simulink model "SOC_Estimation"  (R2022b)
settings: configuration reference "BMS_Sw_CodeGenConfig" (kept outside this file)
undefined symbols (not defined in the file): battery_sli_rtmsupport, BatteryNN, BMS_State_Enum, C1_mat, c_sqrt, DiscIntNeverNeededParam, dV0_mat, gcbh, n, Np_Module, Ns_Module, NumModules, SOCInit, Wc, Wm, x0
libraries: simulink x1
(part 1 of 2)
settings Model: DataDictionary=DD_SOC_Estimation.sldd  ExtModeTrigDuration=5  Creator=cpatel  LastModifiedBy=cpatel
settings ConfigSetRef: SourceName=BMS_Sw_CodeGenConfig

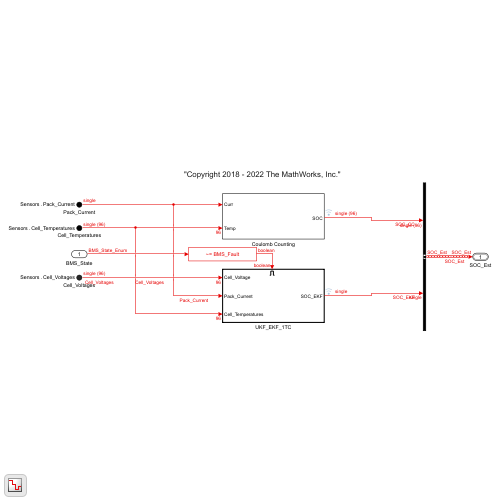
[thumbnail: Simulink's stored preview of the top-level diagram]
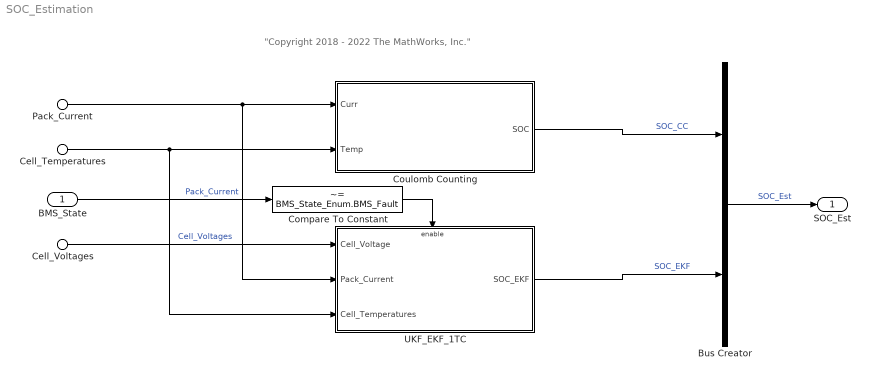
== system SOC_Estimation ==
  note: "Copyright 2018 - 2022 The MathWorks, Inc."
  BMS_State : Inport  OutDataTypeStr=Enum: BMS_State_Enum
  Cell_Voltages : Inport  Port=2  PortName=Sensors  Element=Cell_Voltages
  Pack_Current : Inport  Port=2  PortName=Sensors  Element=Pack_Current
  Cell_Temperatures : Inport  Port=2  PortName=Sensors  Element=Cell_Temperatures
  Bus Creator : BusCreator  Inputs=2  OutDataTypeStr=Bus: SOC_Est  NonVirtualBus=on
      settings: InheritFromInputs=off
  Compare To Constant : simulink/Logic and Bit Operations/Compare To Constant  relop=~=  const=BMS_State_Enum.BMS_Fault  OutDataTypeStr=boolean
  Coulomb Counting : Subsystem  VariantControl=SocAlgo==1
  UKF_EKF_1TC : Subsystem  VariantControl=CellType==1
  SOC_Est : Outport  OutDataTypeStr=Bus: SOC_Est  SampleTime=[0.10000000000000001,0]  VectorParamsAs1DForOutWhenUnconnected=off  BusOutputAsStruct=on
  wires:
  Cell_Voltages/1 -> UKF_EKF_1TC/1(Cell_Voltage)  "Cell_Voltages"
  Bus Creator/1 -> SOC_Est/1  "SOC_Est"
  Coulomb Counting/1(SOC) -> Bus Creator/1  "SOC_CC"
  UKF_EKF_1TC/1(SOC_EKF) -> Bus Creator/2  "SOC_EKF"
  BMS_State/1 -> Compare To Constant/1
  Compare To Constant/1 -> UKF_EKF_1TC/Enable
  Pack_Current/1 -> UKF_EKF_1TC/2(Pack_Current), Coulomb Counting/1(Curr)  "Pack_Current"
  Cell_Temperatures/1 -> Coulomb Counting/2(Temp), UKF_EKF_1TC/3(Cell_Temperatures)

== system SOC_Estimation/Coulomb Counting ==
  Curr : Inport
  Temp : Inport  Port=2
  1-D Lookup Table : Lookup_n-D  NumberOfTableDimensions=1  BreakpointsForDimension1=single(BatteryNN(1).T_vec)  Table=single(BatteryNN(1).AH)*Np_Module  InternalRulePriority=Speed  RndMeth=Simplest
  Discrete-Time Integrator : DiscreteIntegrator  InitialCondition=ones(1,NumModules*Ns_Module)*single(SOCInit)  SampleTime=-1  LimitOutput=on  UpperSaturationLimit=1  LowerSaturationLimit=0  ICPrevOutput=DiscIntNeverNeededParam  ICPrevScaledInput=DiscIntNeverNeededParam
  Divide : Product  Inputs=*/
  Gain : Gain  Gain=single(1/3600)
  SOC : Outport  VectorParamsAs1DForOutWhenUnconnected=off
  wires:
  Discrete-Time Integrator/1 -> SOC/1
  Curr/1 -> Gain/1
  Gain/1 -> Divide/1
  Divide/1 -> Discrete-Time Integrator/1
  1-D Lookup Table/1 -> Divide/2  "Capacity"
  Temp/1 -> 1-D Lookup Table/1

== system SOC_Estimation/UKF_EKF_1TC ==
  note: SOC Blocks have been modified from original library block from Simscape Battery
      | to use Single Data Type
  Cell_Voltage : Inport
  Pack_Current : Inport  Port=2
  Cell_Temperatures : Inport  Port=3
  Enable : EnablePort
  Constant : Constant  Value=single(0.98)
  Constant1 : Constant  Value=single(0.15)
  SOC EKF Estimator (Adaptive Kalman Filter) : Subsystem  LoadFcn=battery_sli_rtmsupport( 'loadfcn', gcbh );  TreatAsAtomicUnit=on  mask(SOC Estimator (Adaptive Kalman Filter)){filterType=Extended Kalman filter, alpha=1, beta=2, kappa=0, Q=|, R=single(0.001), P0=single([1e-2 0 0; 0 1 0; 0 0 1e-8]), Ts=-1, SOC_vec=single(BatteryNN.SOC_vec'), T_vec=single(BatteryNN.T_vec), R1_mat=single(1e-05*ones(11,6)), tau1_mat=single(30*ones(11,6)), V0_mat=single(BatteryNN.V0_mat), AH=single(BatteryNN.AH(1)*Np_Module)}
      mask Q=|
      | single([1e-5 0 0;
      | 0 5e-1 0;0 0 1e-6])
      mask prompts: filterType "physmod:battery:library:comments:control:BatteryEstimators:FilterType_MP"; alpha "physmod:battery:library:comments:control:BatteryEstimators:Alpha_MP"; beta "physmod:battery:library:comments:control:BatteryEstimators:Beta_MP"; kappa "physmod:battery:library:comments:control:BatteryEstimators:Kappa_MP"; Q "physmod:battery:library:comments:control:BatteryEstimators:CovarianceOfTheProcessNoiseQ_MP"; R "physmod:battery:library:comments:control:BatteryEstimators:CovarianceOfTheMeasurementNoiseR_MP"; P0 "physmod:battery:library:comments:control:BatteryEstimators:InitialStateErrorCovarianceP0_MP"; Ts "physmod:battery:library:comments:control:BatteryEstimators:SampleTime1ForInherited_MP"; SOC_vec "physmod:battery:library:comments:control:BatteryEstimators:VectorOfStateofchargeValuesSOC_MP"; T_vec "physmod:battery:library:comments:control:BatteryEstimators:VectorOfTemperaturesT_MP"; R1_mat "physmod:battery:library:comments:control:BatteryEstimators:FirstPolarizationResistanceR1SOCT_MP"; tau1_mat "physmod:battery:library:comments:control:BatteryEstimators:FirstTimeConstantTau1SOCT_MP"; V0_mat "physmod:battery:library:comments:control:BatteryEstimators:NoloadVoltageV0SOCT_MP"; AH "physmod:battery:library:comments:control:BatteryEstimators:CellCapacityAH_MP"
      mask help: physmod:battery:library:comments:control:BatteryEstimators:SOCEstimatorAdaptiveKalmanFilter_MD
      mask init:
      | [C1_mat,dV0_mat,m,n,Wm,Wc,c_sqrt] = battery.mask.initializeKalmanFilter(filterType,tau1_mat,R1_mat,V0_mat,SOC_vec,T_vec,P0,R,Q,alpha,beta,kappa,Ts,AH); %#ok
      settings: CopyFcn=battery_sli_rtmsupport( 'copyfcn', gcbh );  DeleteFcn=battery_sli_rtmsupport( 'deletefcn', gcbh );  ModelCloseFcn=battery_sli_rtmsupport( 'modelclosefcn', gcbh );  PostSaveFcn=battery_sli_rtmsupport( 'postsavefcn', gcbh );  PreCopyFcn=battery_sli_rtmsupport( 'precopyfcn', gcbh );  OpenFcn=battery_sli_rtmsupport( 'openfcn', gcbh );  CloseFcn=battery_sli_rtmsupport( 'closefcn', gcbh );  PreDeleteFcn=battery_sli_rtmsupport( 'predeletefcn', gcbh );
      settings: LibrarySourceBlock=|
      | batt_sl_lib/Estimators/SOC Estimator
      | (Adaptive Kalman Filter)
      mask Help: web(nesl_help(gcbh))
      mask TypeOptions filterType: Kalman Filter/filterType
      mask Callback filterType: battery.mask.callbackPopupKalmanFilter(gcb);
      mask DialogControl Container6 Prompt: physmod:battery:library:comments:control:BatteryEstimators:tab_Main
      mask DialogControl filterType Prompt: Filter type
      mask DialogControl alpha Prompt: Alpha
      mask DialogControl beta Prompt: Beta
      mask DialogControl kappa Prompt: Kappa
      mask DialogControl Q Prompt: Covariance of the process noise, Q
      mask DialogControl R Prompt: Covariance of the measurement noise, R
      mask DialogControl P0 Prompt: Initial state error covariance, P0
      mask DialogControl Ts Prompt: Sample time (-1 for inherited)
      mask DialogControl Container4 Prompt: physmod:battery:library:comments:control:BatteryEstimators:tab_SystemModel
      mask DialogControl SOC_vec Prompt: Vector of state-of-charge values, SOC (-)
      mask DialogControl T_vec Prompt: Vector of temperatures, T
      mask DialogControl R1_mat Prompt: First polarization resistance, R1(SOC,T), (ohm)
      mask DialogControl tau1_mat Prompt: First time constant, tau1(SOC,T), (s)
      mask DialogControl V0_mat Prompt: No-load voltage, V0(SOC,T), (V)
      mask DialogControl AH Prompt: Cell capacity, AH (A*Hr)
  Selector : Selector  InputPortWidth=Ns_Module*NumModules  IndexOptions=Starting index (dialog)  Indices=[1]  OutputSizes=1
  Selector1 : Selector  InputPortWidth=Ns_Module*NumModules  IndexOptions=Starting index (dialog)  Indices=[1]  OutputSizes=1
  Terminator1 : Terminator
  SOC_EKF : Outport  VectorParamsAs1DForOutWhenUnconnected=off
  wires:
  Pack_Current/1 -> SOC EKF Estimator (Adaptive Kalman Filter)/1(PackCurrent)  "PackCurrent"
  SOC EKF Estimator (Adaptive Kalman Filter)/2(R0) -> Terminator1/1
  Cell_Temperatures/1 -> Selector1/1
  Cell_Voltage/1 -> Selector/1
  SOC EKF Estimator (Adaptive Kalman Filter)/1(SOC) -> SOC_EKF/1
  Selector/1 -> SOC EKF Estimator (Adaptive Kalman Filter)/2(CellVoltage)
  Selector1/1 -> SOC EKF Estimator (Adaptive Kalman Filter)/3(CellTemperature)
  Constant/1 -> SOC EKF Estimator (Adaptive Kalman Filter)/4(InitialSOC)
  Constant1/1 -> SOC EKF Estimator (Adaptive Kalman Filter)/5(InitialR0)

== system SOC_Estimation/UKF_EKF_1TC/SOC EKF Estimator (Adaptive Kalman Filter) ==
  PackCurrent : Inport
  CellVoltage : Inport  Port=2  Partition=on  PartitionDimension=1  PartitionWidth=1  PartitionOffset=0
  CellTemperature : Inport  Port=3  Partition=on  PartitionDimension=1  PartitionWidth=1  PartitionOffset=0
  InitialSOC : Inport  Port=4  Partition=on  PartitionDimension=1  PartitionWidth=1  PartitionOffset=0
  InitialR0 : Inport  Port=5  Partition=on  PartitionDimension=1  PartitionWidth=1  PartitionOffset=0
  For Each : ForEach  DisableCoverage=on  IterateSubsysMaskParameter=off,off,off,off,off,off,off,off,off,off,off,off,off,off
  Gain : Gain  Gain=-1
  Kalman Filter : Subsystem  Variant=on  VariantControlMode=label  VariantControl=Choice  LabelModeActiveChoice=EKF  mask{filterType=Extended Kalman filter}
      mask prompts: filterType "Filter type"
      mask TypeOptions filterType: physmod:battery:library:comments:control:BatteryEstimators:ExtendedKalmanFilter_PV | physmod:battery:library:comments:control:BatteryEstimators:ExtendedKalmanBucyFilter_PV | physmod:battery:library:comments:control:BatteryEstimators:UnscentedKalmanFilter_PV | physmod:battery:library:comments:control:BatteryEstimators:UnscentedKalmanBucyFilter_PV
      mask Callback filterType: battery.mask.callbackTypeKalmanFilter(gcb)
  Selector : Selector  InputPortWidth=3  IndexOptions=Index vector (dialog)  Indices=1  OutputSizes=1
  Selector1 : Selector  InputPortWidth=3  IndexOptions=Index vector (dialog)  Indices=3  OutputSizes=1
  SOC : Outport  ConcatenationDimension=1
  R0 : Outport  Port=2  ConcatenationDimension=1
  wires:
  Gain/1 -> Kalman Filter/2(PackCurrent)
  InitialR0/1 -> Kalman Filter/5(InitialR0)
  InitialSOC/1 -> Kalman Filter/4(InitialSOC)
  CellTemperature/1 -> Kalman Filter/3(CellTemperature)
  PackCurrent/1 -> Gain/1
  CellVoltage/1 -> Kalman Filter/1(CellVoltage)
  Selector1/1 -> R0/1
  Selector/1 -> SOC/1
  Kalman Filter/1(xhat) -> Selector1/1, Selector/1

== system SOC_Estimation/UKF_EKF_1TC/SOC EKF Estimator (Adaptive Kalman Filter)/Kalman Filter ==
  CellVoltage : Inport
  PackCurrent : Inport  Port=2
  CellTemperature : Inport  Port=3
  InitialSOC : Inport  Port=4
  InitialR0 : Inport  Port=5
  EKBF : Subsystem  VariantControl=EKBF
  EKF : Subsystem  VariantControl=EKF
  UKBF : Subsystem  VariantControl=UKBF
  UKF : Subsystem  VariantControl=UKF
  xhat : Outport

== system SOC_Estimation/UKF_EKF_1TC/SOC EKF Estimator (Adaptive Kalman Filter)/Kalman Filter/EKBF ==
  CellVoltage : Inport
  PackCurrent : Inport  Port=2
  CellTemperature : Inport  Port=3
  InitialSOC : Inport  Port=4
  InitialR0 : Inport  Port=5
  Jacobian : Subsystem
  Prediction-correction : Subsystem
      settings: PortSchema="{\"entries\":[{\"content\":{\"sides\":[{\"content\":{\"connectorIds\":[\"In1\",\"In2\",\"In3\",\"In4\",\"In5\"]},\"type\":\"ConnectorPlacement.EquallySpacedRectSide\",\"uuid\":\"70763294-f6a8-4957-b17c-9720b328d616\"},{\"content\":{\"connectorIds\":[\"Out1\"],\"side\":\"RIGHT\"},\"type\":\"ConnectorPlacement.EquallySpacedRectSide\",\"uuid\":\"9ab31a02-4943-4cb5-b23b-ea78b251bb22\"},{\"content\":{\"connectorIds\":[\"In6\"],\"side\":\"TOP\"},\"type\":\"ConnectorPlacement.EquallySpacedRectSide\",\"uuid\":\"49dcdbdb-b164-4a45-b3b9-2ea25dc0ed02\"}]},\"type\":\"ConnectorPlacement.EquallySpacedConnector\",\"uuid\":\"ec3a5245-b8fb-46be-bfec-cf80f908588d\"}],\"packageUris\":[\"http://schema.mathworks.com/mf0/Connector/R2020b\"],\"version\":\"1.0\"}"
  Reshape : Reshape
  Sum : Sum  Inputs=|+-
  xhat : Outport
  wires:
  Reshape/1 -> xhat/1
  InitialR0/1 -> Prediction-correction/5(InitialR0)
  InitialSOC/1 -> Prediction-correction/4(InitialSOC)
  CellTemperature/1 -> Jacobian/2(Temperature)
  PackCurrent/1 -> Jacobian/1(current)
  CellVoltage/1 -> Sum/1
  Jacobian/2(f(x)) -> Prediction-correction/1(f(x))
  Jacobian/1(Vt_model) -> Sum/2
  Prediction-correction/1(x) -> Jacobian/3(x), Reshape/1
  Sum/1 -> Prediction-correction/6(Vt_error)
  Jacobian/3(F) -> Prediction-correction/2(F)
  Jacobian/4(H) -> Prediction-correction/3(H)

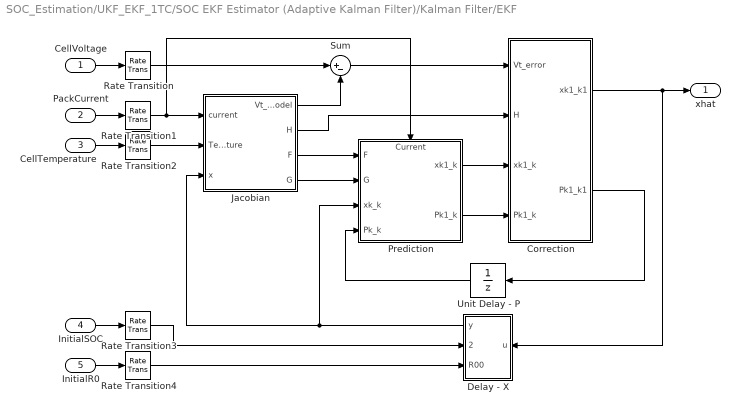
== system SOC_Estimation/UKF_EKF_1TC/SOC EKF Estimator (Adaptive Kalman Filter)/Kalman Filter/EKF ==
  CellVoltage : Inport
  PackCurrent : Inport  Port=2
  CellTemperature : Inport  Port=3
  InitialSOC : Inport  Port=4
  InitialR0 : Inport  Port=5
  Correction : Subsystem
  Delay - X : Subsystem
      settings: PortSchema="{\"entries\":[{\"content\":{\"sides\":[{\"content\":{\"connectorIds\":[\"In1\"]},\"type\":\"ConnectorPlacement.EquallySpacedRectSide\",\"uuid\":\"400f522a-a807-4994-87ff-7e153ef60805\"},{\"content\":{\"connectorIds\":[\"Out1\",\"In2\",\"In3\"],\"side\":\"RIGHT\"},\"type\":\"ConnectorPlacement.EquallySpacedRectSide\",\"uuid\":\"6cda2f6d-d263-4e07-9a58-81074bd43172\"},{\"content\":{\"connectorIds\":[],\"side\":\"TOP\"},\"type\":\"ConnectorPlacement.EquallySpacedRectSide\",\"uuid\":\"9ba66b88-6997-492b-8290-d222d6d8f8af\"}]},\"type\":\"ConnectorPlacement.EquallySpacedConnector\",\"uuid\":\"f2f17bef-02dc-403f-b8af-5b97399a5e6c\"}],\"packageUris\":[\"http://schema.mathworks.com/mf0/Connector/R2020b\"],\"version\":\"1.0\"}"
  Jacobian : Subsystem
  Prediction : Subsystem
      settings: PortSchema="{\"entries\":[{\"content\":{\"sides\":[{\"content\":{\"connectorIds\":[\"In1\",\"In2\",\"In3\",\"In4\"]},\"type\":\"ConnectorPlacement.EquallySpacedRectSide\",\"uuid\":\"769ad24d-2d7f-40f9-a049-32dd41bae35d\"},{\"content\":{\"connectorIds\":[\"Out1\",\"Out2\"],\"side\":\"RIGHT\"},\"type\":\"ConnectorPlacement.EquallySpacedRectSide\",\"uuid\":\"b91eca28-d625-4904-9292-6163fd48fb7b\"},{\"content\":{\"connectorIds\":[\"In5\"],\"side\":\"TOP\"},\"type\":\"ConnectorPlacement.EquallySpacedRectSide\",\"uuid\":\"03f245fa-72f0-4cdc-a162-c307173ac60c\"}]},\"type\":\"ConnectorPlacement.EquallySpacedConnector\",\"uuid\":\"70aef080-af31-4b50-8c38-7ffc1907abe4\"}],\"packageUris\":[\"http://schema.mathworks.com/mf0/Connector/R2020b\"],\"version\":\"1.0\"}"
  Rate Transition{,1..4} (5 alike) : RateTransition  OutPortSampleTime=Ts
  Sum : Sum  Inputs=|+-
  Unit Delay - P : UnitDelay  InitialCondition=P0  SampleTime=Ts  HasFrameUpgradeWarning=on
  xhat : Outport
  wires:
  Rate Transition4/1 -> Delay - X/3(R00)
  Rate Transition3/1 -> Delay - X/2(SOC0)
  InitialR0/1 -> Rate Transition4/1
  InitialSOC/1 -> Rate Transition3/1
  Rate Transition2/1 -> Jacobian/2(Temperature)
  Rate Transition1/1 -> Prediction/5(Current), Jacobian/1(current)
  Rate Transition/1 -> Sum/1
  Prediction/2(Pk1_k) -> Correction/4(Pk1_k)
  CellVoltage/1 -> Rate Transition/1
  Jacobian/2(H) -> Correction/2(H)
  Prediction/1(xk1_k) -> Correction/3(xk1_k)
  CellTemperature/1 -> Rate Transition2/1
  Sum/1 -> Correction/1(Vt_error)
  Jacobian/4(G) -> Prediction/2(G)
  Jacobian/1(Vt_model) -> Sum/2
  Correction/1(xk1_k1) -> xhat/1, Delay - X/1(u)
  Jacobian/3(F) -> Prediction/1(F)
  Correction/2(Pk1_k1) -> Unit Delay - P/1
  PackCurrent/1 -> Rate Transition1/1
  Delay - X/1(y) -> Prediction/3(xk_k), Jacobian/3(x)
  Unit Delay - P/1 -> Prediction/4(Pk_k)

== system SOC_Estimation/UKF_EKF_1TC/SOC EKF Estimator (Adaptive Kalman Filter)/Kalman Filter/UKBF ==
  CellVoltage : Inport
  PackCurrent : Inport  Port=2
  CellTemperature : Inport  Port=3
  InitialSOC : Inport  Port=4
  InitialR0 : Inport  Port=5
  Constant : Constant  Value=chol(P0,'lower')
  Constant1 : Constant  Value=0
  Mux : Mux  Inputs=3
  Prediction-correction : Subsystem
  Reshape : Reshape  OutputDimensionality=Customize  OutputDimensions=[n,1]
  Reshape1 : Reshape
  Sigma points init : Subsystem
  xhat : Outport
  wires:
  Reshape1/1 -> xhat/1
  Reshape/1 -> Sigma points init/1(x0)
  Constant1/1 -> Mux/2
  InitialR0/1 -> Mux/3
  InitialSOC/1 -> Mux/1
  CellVoltage/1 -> Prediction-correction/3(Voltage)
  CellTemperature/1 -> Prediction-correction/2(Temperature)
  PackCurrent/1 -> Prediction-correction/1(Current)
  Prediction-correction/1(xhat) -> Reshape1/1
  Sigma points init/1(X0) -> Prediction-correction/4(X0)
  Constant/1 -> Sigma points init/2(A)
  Mux/1 -> Reshape/1

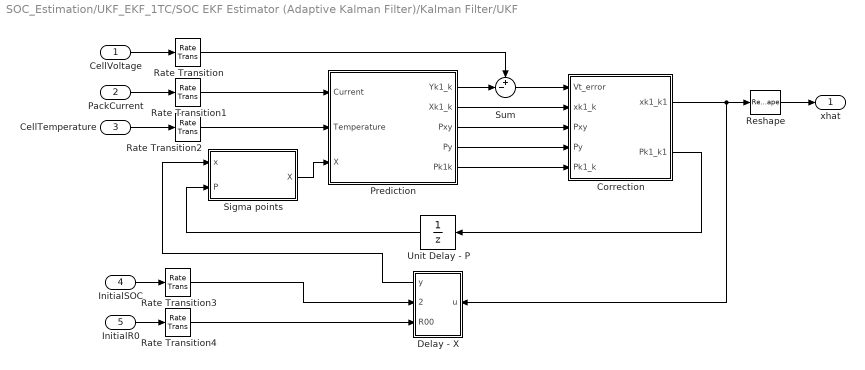
== system SOC_Estimation/UKF_EKF_1TC/SOC EKF Estimator (Adaptive Kalman Filter)/Kalman Filter/UKF ==
  CellVoltage : Inport
  PackCurrent : Inport  Port=2
  CellTemperature : Inport  Port=3
  InitialSOC : Inport  Port=4
  InitialR0 : Inport  Port=5
  Correction : Subsystem
  Delay - X : Subsystem
      settings: PortSchema="{\"entries\":[{\"content\":{\"sides\":[{\"content\":{\"connectorIds\":[\"In1\"]},\"type\":\"ConnectorPlacement.EquallySpacedRectSide\",\"uuid\":\"400f522a-a807-4994-87ff-7e153ef60805\"},{\"content\":{\"connectorIds\":[\"Out1\",\"In2\",\"In3\"],\"side\":\"RIGHT\"},\"type\":\"ConnectorPlacement.EquallySpacedRectSide\",\"uuid\":\"6cda2f6d-d263-4e07-9a58-81074bd43172\"},{\"content\":{\"connectorIds\":[],\"side\":\"TOP\"},\"type\":\"ConnectorPlacement.EquallySpacedRectSide\",\"uuid\":\"9ba66b88-6997-492b-8290-d222d6d8f8af\"}]},\"type\":\"ConnectorPlacement.EquallySpacedConnector\",\"uuid\":\"f2f17bef-02dc-403f-b8af-5b97399a5e6c\"}],\"packageUris\":[\"http://schema.mathworks.com/mf0/Connector/R2020b\"],\"version\":\"1.0\"}"
  Prediction : Subsystem
  Rate Transition{,1..4} (5 alike) : RateTransition  OutPortSampleTime=Ts
  Reshape : Reshape
  Sigma points : Subsystem
  Sum : Sum  Inputs=+-|
  Unit Delay - P : UnitDelay  InitialCondition=chol(P0,'lower')  SampleTime=Ts  HasFrameUpgradeWarning=on
  xhat : Outport
  wires:
  Rate Transition4/1 -> Delay - X/3(R00)
  Rate Transition3/1 -> Delay - X/2(SOC0)
  InitialSOC/1 -> Rate Transition3/1
  InitialR0/1 -> Rate Transition4/1
  Rate Transition2/1 -> Prediction/2(Temperature)
  Rate Transition1/1 -> Prediction/1(Current)
  Rate Transition/1 -> Sum/1
  Reshape/1 -> xhat/1
  Prediction/2(Xk1_k) -> Correction/2(xk1_k)
  Correction/2(Pk1_k1) -> Unit Delay - P/1
  Correction/1(xk1_k1) -> Reshape/1, Delay - X/1(u)
  Unit Delay - P/1 -> Sigma points/2(P)
  Prediction/3(Pxy) -> Correction/3(Pxy)
  Prediction/4(Py) -> Correction/4(Py)
  CellTemperature/1 -> Rate Transition2/1
  Sigma points/1(X) -> Prediction/3(X)
  Sum/1 -> Correction/1(Vt_error)
  Delay - X/1(y) -> Sigma points/1(x)
  PackCurrent/1 -> Rate Transition1/1
  Prediction/5(Pk1k) -> Correction/5(Pk1_k)
  CellVoltage/1 -> Rate Transition/1
  Prediction/1(Yk1_k) -> Sum/2

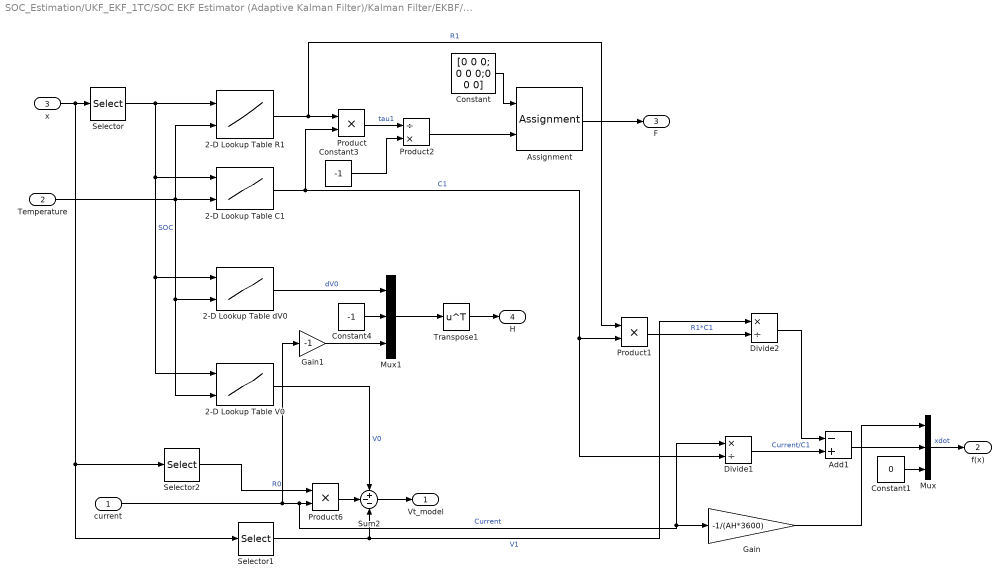
== system SOC_Estimation/UKF_EKF_1TC/SOC EKF Estimator (Adaptive Kalman Filter)/Kalman Filter/EKBF/Jacobian ==
  current : Inport
  Temperature : Inport  Port=2
  x : Inport  Port=3
  2-D Lookup Table C1 : Lookup_n-D  BreakpointsForDimension1=SOC_vec  BreakpointsForDimension2=T_vec  Table=C1_mat  InternalRulePriority=Speed  RndMeth=Simplest
      settings: InputPortMap=u0,u1
  2-D Lookup Table R1 : Lookup_n-D  BreakpointsForDimension1=SOC_vec  BreakpointsForDimension2=T_vec  Table=R1_mat  InternalRulePriority=Speed  RndMeth=Simplest
      settings: InputPortMap=u0,u1
  2-D Lookup Table V0 : Lookup_n-D  BreakpointsForDimension1=SOC_vec  BreakpointsForDimension2=T_vec  Table=V0_mat  InternalRulePriority=Speed  RndMeth=Simplest
      settings: InputPortMap=u0,u1
  2-D Lookup Table dV0 : Lookup_n-D  BreakpointsForDimension1=SOC_vec  BreakpointsForDimension2=T_vec  Table=dV0_mat  InternalRulePriority=Speed  RndMeth=Simplest
      settings: InputPortMap=u0,u1
  Add1 : Sum  Inputs=-+
  Assignment : Assignment  NumberOfDimensions=2  DiagnosticForDimensions=Warning  IndexOptions=Index vector (dialog),Index vector (dialog)  Indices=2,2  OutputSizes=1,1
  Constant : Constant  Value=|
      | [0 0 0;
      | 0 0 0;0 0 0]
  Constant1 : Constant  Value=0
  Constant3 : Constant  Value=-1
  Constant4 : Constant  Value=-1
  Divide1 : Product  Inputs=*/
  Divide2 : Product  Inputs=*/
  Gain : Gain  Gain=-1/(AH*3600)
  Gain1 : Gain  Gain=-1
  Mux : Mux  Inputs=3
  Mux1 : Mux  Inputs=3
  Product : Product
  Product1 : Product
  Product2 : Product  Inputs=/*
  Product6 : Product
  Selector : Selector  InputPortWidth=3  IndexOptions=Index vector (dialog)  Indices=1  OutputSizes=1
  Selector1 : Selector  InputPortWidth=3  IndexOptions=Index vector (dialog)  Indices=2  OutputSizes=1
  Selector2 : Selector  InputPortWidth=3  IndexOptions=Index vector (dialog)  Indices=3  OutputSizes=1
  Sum2 : Sum  Inputs=+--
  Transpose1 : Math  Operator=transpose
  Vt_model : Outport
  f(x) : Outport  Port=2
  F : Outport  Port=3
  H : Outport  Port=4
  wires:
  Constant1/1 -> Mux/3
  Gain1/1 -> Mux1/3
  Divide2/1 -> Add1/1
  Gain/1 -> Mux/1
  current/1 -> Gain/1, Divide1/1, Product6/2, Gain1/1  "Current"
  Add1/1 -> Mux/2
  2-D Lookup Table R1/1 -> Product/1, Product1/1  "R1"
  2-D Lookup Table C1/1 -> Product/2, Divide1/2, Product1/2  "C1"
  Product1/1 -> Divide2/2  "R1*C1"
  Mux/1 -> f(x)/1  "xdot"
  Divide1/1 -> Add1/2  "Current/C1"
  2-D Lookup Table dV0/1 -> Mux1/1  "dV0"
  Constant4/1 -> Mux1/2
  Transpose1/1 -> H/1
  Mux1/1 -> Transpose1/1
  x/1 -> Selector/1, Selector1/1, Selector2/1
  Temperature/1 -> 2-D Lookup Table R1/2, 2-D Lookup Table C1/2, 2-D Lookup Table V0/2, 2-D Lookup Table dV0/2
  Selector/1 -> 2-D Lookup Table R1/1, 2-D Lookup Table V0/1, 2-D Lookup Table dV0/1, 2-D Lookup Table C1/1  "SOC"
  Constant/1 -> Assignment/1
  Product2/1 -> Assignment/2
  Assignment/1 -> F/1
  Constant3/1 -> Product2/2
  Selector2/1 -> Product6/1  "R0"
  Product6/1 -> Sum2/2
  Selector1/1 -> Sum2/3, Divide2/1  "V1"
  Sum2/1 -> Vt_model/1
  2-D Lookup Table V0/1 -> Sum2/1  "V0"
  Product/1 -> Product2/1  "tau1"

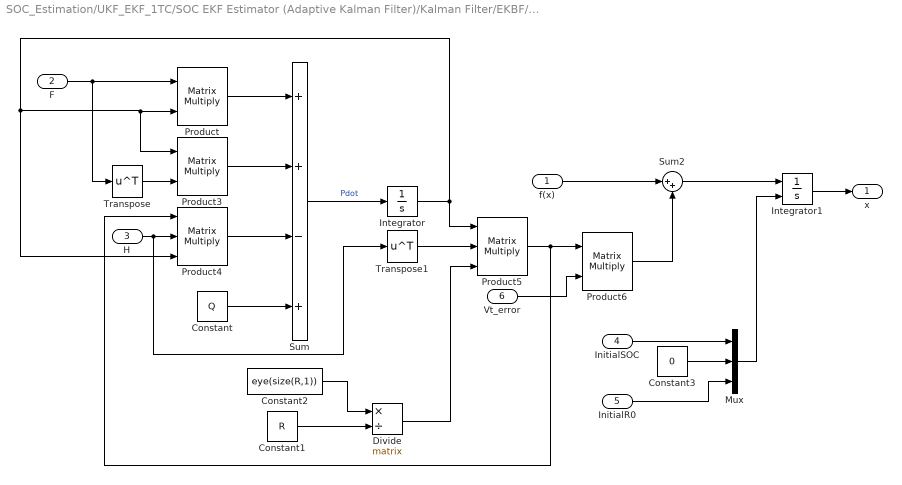
== system SOC_Estimation/UKF_EKF_1TC/SOC EKF Estimator (Adaptive Kalman Filter)/Kalman Filter/EKBF/Prediction-correction ==
  f(x) : Inport
  F : Inport  Port=2
  H : Inport  Port=3
  InitialSOC : Inport  Port=4
  InitialR0 : Inport  Port=5
  Vt_error : Inport  Port=6
  Constant : Constant  Value=Q
  Constant1 : Constant  Value=R
  Constant2 : Constant  Value=eye(size(R,1))
  Constant3 : Constant  Value=0
  Divide : Product  Inputs=*/  Multiplication=Matrix(*)
  Integrator : Integrator  InitialCondition=P0
  Integrator1 : Integrator  InitialConditionSource=external  InitialCondition=x0
  Mux : Mux  Inputs=3
  Product : Product  Multiplication=Matrix(*)
  Product3 : Product  Multiplication=Matrix(*)
  Product4 : Product  Inputs=3  Multiplication=Matrix(*)
  Product5 : Product  Inputs=3  Multiplication=Matrix(*)
  Product6 : Product  Multiplication=Matrix(*)
  Sum : Sum  Inputs=++-+
  Sum2 : Sum  Inputs=|++
  Transpose : Math  Operator=transpose
  Transpose1 : Math  Operator=transpose
  x : Outport
  wires:
  Constant3/1 -> Mux/2
  InitialR0/1 -> Mux/3
  InitialSOC/1 -> Mux/1
  Mux/1 -> Integrator1/2
  Integrator/1 -> Product3/1, Product/2, Product4/3, Product5/1
  Product/1 -> Sum/1
  Product3/1 -> Sum/2
  Transpose/1 -> Product3/2
  Product4/1 -> Sum/3
  Constant/1 -> Sum/4
  Sum/1 -> Integrator/1  "Pdot"
  Transpose1/1 -> Product5/2
  Constant1/1 -> Divide/2
  Divide/1 -> Product5/3
  Constant2/1 -> Divide/1
  Product5/1 -> Product4/1, Product6/1
  Integrator1/1 -> x/1
  F/1 -> Product/1, Transpose/1
  H/1 -> Transpose1/1, Product4/2
  Vt_error/1 -> Product6/2
  Product6/1 -> Sum2/2
  Sum2/1 -> Integrator1/1
  f(x)/1 -> Sum2/1

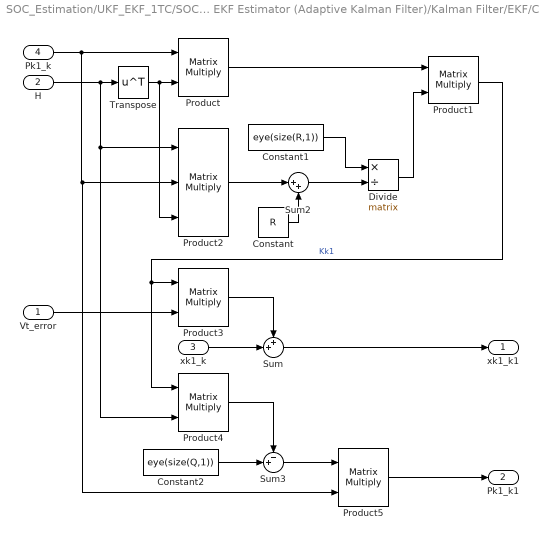
== system SOC_Estimation/UKF_EKF_1TC/SOC EKF Estimator (Adaptive Kalman Filter)/Kalman Filter/EKF/Correction ==
  Vt_error : Inport
  H : Inport  Port=2
  xk1_k : Inport  Port=3
  Pk1_k : Inport  Port=4
  Constant : Constant  Value=R
  Constant1 : Constant  Value=eye(size(R,1))  OutDataTypeStr=Inherit: Inherit via back propagation
  Constant2 : Constant  Value=eye(size(Q,1))  OutDataTypeStr=Inherit: Inherit via back propagation
  Divide : Product  Inputs=*/  Multiplication=Matrix(*)
  Product{,1,3..5} (5 alike) : Product  Multiplication=Matrix(*)
  Product2 : Product  Inputs=3  Multiplication=Matrix(*)
  Sum : Sum  Inputs=++|
  Sum2 : Sum  Inputs=|++
  Sum3 : Sum  Inputs=-+|
  Transpose : Math  Operator=transpose
  xk1_k1 : Outport
  Pk1_k1 : Outport  Port=2
  wires:
  H/1 -> Product4/2, Product2/1, Transpose/1
  Transpose/1 -> Product2/3, Product/2
  Pk1_k/1 -> Product5/2, Product2/2, Product/1
  Product/1 -> Product1/1
  Product2/1 -> Sum2/1
  Constant/1 -> Sum2/2
  Product1/1 -> Product3/1, Product4/1  "Kk1"
  Sum2/1 -> Divide/2
  Divide/1 -> Product1/2
  Constant1/1 -> Divide/1
  xk1_k/1 -> Sum/2
  Vt_error/1 -> Product3/2
  Product3/1 -> Sum/1
  Sum/1 -> xk1_k1/1
  Constant2/1 -> Sum3/2
  Product4/1 -> Sum3/1
  Sum3/1 -> Product5/1
  Product5/1 -> Pk1_k1/1

== system SOC_Estimation/UKF_EKF_1TC/SOC EKF Estimator (Adaptive Kalman Filter)/Kalman Filter/EKF/Delay - X ==
  u : Inport
  SOC0 : Inport  Port=2
  R00 : Inport  Port=3
  Constant1 : Constant  Value=0  OutDataTypeStr=Inherit: Inherit via back propagation
  Delay : Delay  DelayLength=1  InitialConditionSource=Input port  SampleTime=Ts
      settings: InputPortMap=u0,p4
  Mux : Mux  Inputs=3
  y : Outport
  wires:
  R00/1 -> Mux/3
  u/1 -> Delay/1
  Delay/1 -> y/1
  Mux/1 -> Delay/2
  SOC0/1 -> Mux/1
  Constant1/1 -> Mux/2

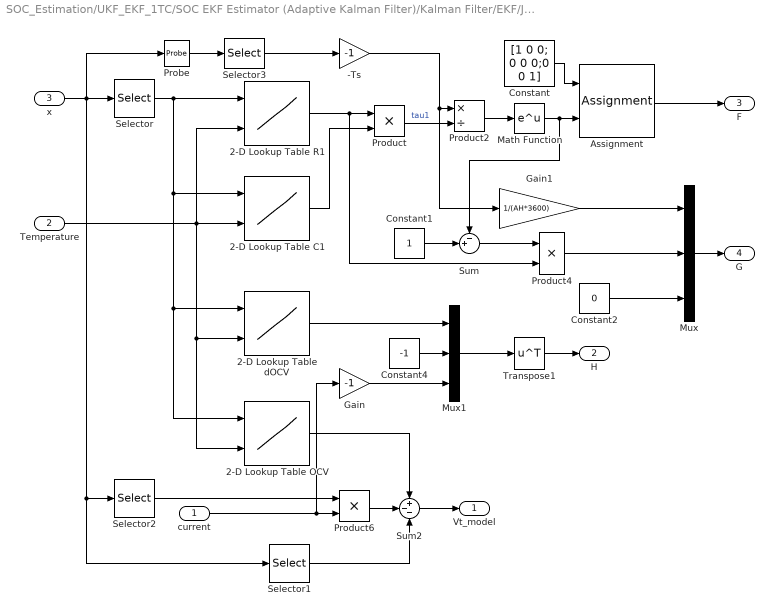
== system SOC_Estimation/UKF_EKF_1TC/SOC EKF Estimator (Adaptive Kalman Filter)/Kalman Filter/EKF/Jacobian ==
  current : Inport
  Temperature : Inport  Port=2
  x : Inport  Port=3
  -Ts : Gain  Gain=-1
  2-D Lookup Table C1 : Lookup_n-D  BreakpointsForDimension1=SOC_vec  BreakpointsForDimension2=T_vec  Table=C1_mat  InternalRulePriority=Speed  RndMeth=Simplest
      settings: InputPortMap=u0,u1
  2-D Lookup Table OCV : Lookup_n-D  BreakpointsForDimension1=SOC_vec  BreakpointsForDimension2=T_vec  Table=V0_mat  InternalRulePriority=Speed  RndMeth=Simplest
      settings: InputPortMap=u0,u1
  2-D Lookup Table R1 : Lookup_n-D  BreakpointsForDimension1=SOC_vec  BreakpointsForDimension2=T_vec  Table=R1_mat  InternalRulePriority=Speed  RndMeth=Simplest
      settings: InputPortMap=u0,u1
  2-D Lookup Table dOCV : Lookup_n-D  BreakpointsForDimension1=SOC_vec  BreakpointsForDimension2=T_vec  Table=dV0_mat  InternalRulePriority=Speed  RndMeth=Simplest
      settings: InputPortMap=u0,u1
  Assignment : Assignment  NumberOfDimensions=2  DiagnosticForDimensions=Warning  IndexOptions=Index vector (dialog),Index vector (dialog)  Indices=2,2  OutputSizes=1,1
  Constant : Constant  Value=|  OutDataTypeStr=Inherit: Inherit via back propagation
      | [1 0 0;
      | 0 0 0;0 0 1]
  Constant1 : Constant  OutDataTypeStr=Inherit: Inherit via back propagation
  Constant2 : Constant  Value=0  OutDataTypeStr=Inherit: Inherit via back propagation
  Constant4 : Constant  Value=-1  OutDataTypeStr=Inherit: Inherit via back propagation
  Gain : Gain  Gain=-1
  Gain1 : Gain  Gain=1/(AH*3600)
  Math Function : Math
  Mux : Mux  Inputs=3
  Mux1 : Mux  Inputs=3
  Probe : Probe  ProbeWidth=off  ProbeComplexSignal=off  ProbeSampleTimeDataType=single
  Product : Product
  Product2 : Product  Inputs=*/
  Product4 : Product
  Product6 : Product
  Selector : Selector  InputPortWidth=3  IndexOptions=Index vector (dialog)  Indices=1  OutputSizes=1
  Selector1 : Selector  InputPortWidth=3  IndexOptions=Index vector (dialog)  Indices=2  OutputSizes=1
  Selector2 : Selector  InputPortWidth=3  IndexOptions=Index vector (dialog)  Indices=3  OutputSizes=1
  Selector3 : Selector  InputPortWidth=2  IndexOptions=Index vector (dialog)  Indices=1  OutputSizes=1
  Sum : Sum  Inputs=-+|
  Sum2 : Sum  Inputs=+--
  Transpose1 : Math  Operator=transpose
  Vt_model : Outport
  H : Outport  Port=2
  F : Outport  Port=3
  G : Outport  Port=4
  wires:
  Selector3/1 -> -Ts/1
  Probe/1 -> Selector3/1
  Constant2/1 -> Mux/3
  Gain/1 -> Mux1/3
  current/1 -> Product6/2, Gain/1
  Temperature/1 -> 2-D Lookup Table OCV/2, 2-D Lookup Table dOCV/2, 2-D Lookup Table C1/2, 2-D Lookup Table R1/2
  Selector/1 -> 2-D Lookup Table R1/1, 2-D Lookup Table C1/1, 2-D Lookup Table OCV/1, 2-D Lookup Table dOCV/1
  x/1 -> Selector1/1, Selector2/1, Selector/1, Probe/1
  Constant/1 -> Assignment/1
  Math Function/1 -> Assignment/2, Sum/1
  2-D Lookup Table R1/1 -> Product4/2, Product/1
  2-D Lookup Table C1/1 -> Product/2
  Product/1 -> Product2/2  "tau1"
  Product2/1 -> Math Function/1
  Assignment/1 -> F/1
  Constant1/1 -> Sum/2
  Sum/1 -> Product4/1
  -Ts/1 -> Product2/1, Gain1/1
  Product4/1 -> Mux/2
  Mux/1 -> G/1
  Constant4/1 -> Mux1/2
  Selector2/1 -> Product6/1
  Product6/1 -> Sum2/2
  Selector1/1 -> Sum2/3
  Mux1/1 -> Transpose1/1
  Transpose1/1 -> H/1
  Sum2/1 -> Vt_model/1
  2-D Lookup Table OCV/1 -> Sum2/1
  2-D Lookup Table dOCV/1 -> Mux1/1
  Gain1/1 -> Mux/1

== system SOC_Estimation/UKF_EKF_1TC/SOC EKF Estimator (Adaptive Kalman Filter)/Kalman Filter/EKF/Prediction ==
  F : Inport
  G : Inport  Port=2
  xk_k : Inport  Port=3
  Pk_k : Inport  Port=4
  Current : Inport  Port=5
  Constant : Constant  Value=Q  OutDataTypeStr=Inherit: Inherit via back propagation
  Product : Product  Multiplication=Matrix(*)
  Product1 : Product  Multiplication=Matrix(*)
  Product2 : Product  Inputs=3  Multiplication=Matrix(*)
  Sum : Sum  Inputs=|++
  Sum1 : Sum  Inputs=|++
  Transpose : Math  Operator=transpose
  xk1_k : Outport
  Pk1_k : Outport  Port=2
  wires:
  F/1 -> Transpose/1, Product2/1, Product/1
  xk_k/1 -> Product/2
  G/1 -> Product1/1
  Current/1 -> Product1/2
  Product/1 -> Sum/1
  Product1/1 -> Sum/2
  Sum/1 -> xk1_k/1
  Pk_k/1 -> Product2/2
  Transpose/1 -> Product2/3
  Product2/1 -> Sum1/1
  Constant/1 -> Sum1/2
  Sum1/1 -> Pk1_k/1

== system SOC_Estimation/UKF_EKF_1TC/SOC EKF Estimator (Adaptive Kalman Filter)/Kalman Filter/UKBF/Prediction-correction ==
  Current : Inport
  Temperature : Inport  Port=2
  Voltage : Inport  Port=3
  X0 : Inport  Port=4
  Integrator1 : Integrator  InitialConditionSource=external
  Measurement function : Subsystem  TreatAsAtomicUnit=on
  State function : Subsystem  TreatAsAtomicUnit=on
  Sum of Elements : Sum  Inputs=+  CollapseMode=Specified dimension  CollapseDim=2
  Sum of Elements1 : Sum  Inputs=+  CollapseMode=Specified dimension  CollapseDim=2
  Sum of Elements2 : Sum  Inputs=+  CollapseMode=Specified dimension  CollapseDim=2
  Update A : Subsystem
  Xdot : Subsystem
  xhat : Outport
  wires:
  Sum of Elements2/1 -> Xdot/5(mf)
  Integrator1/1 -> Update A/1(X), Xdot/7(X), Measurement function/3(X), State function/3(X)
  Sum of Elements1/1 -> Xdot/6(mx)
  Sum of Elements/1 -> Xdot/3(mh)
  State function/3(mx) -> Sum of Elements1/1
  State function/2(mf) -> Sum of Elements2/1
  Measurement function/2(mh) -> Sum of Elements/1
  Xdot/1(Xdot) -> Integrator1/1
  Update A/1(A(t)) -> Xdot/8(A)
  Update A/2(xhat) -> xhat/1
  Temperature/1 -> Measurement function/2(Temperature), State function/2(Temperature)
  Current/1 -> Measurement function/1(Current), State function/1(Current)
  X0/1 -> Integrator1/2
  State function/1(f(X)) -> Xdot/4(f(X))
  Measurement function/1(h(X)) -> Xdot/2(h(X))
  Voltage/1 -> Xdot/1(Voltage)

== system SOC_Estimation/UKF_EKF_1TC/SOC EKF Estimator (Adaptive Kalman Filter)/Kalman Filter/UKBF/Sigma points init ==
  x0 : Inport
  A : Inport  Port=2
  Assignment : Assignment  NumberOfDimensions=2  DiagnosticForDimensions=Warning  IndexOptions=Index vector (dialog),Index vector (dialog)  Indices=1:n,1  OutputSizes=1,1
  Assignment1 : Assignment  NumberOfDimensions=2  DiagnosticForDimensions=Warning  IndexOptions=Index vector (dialog),Index vector (dialog)  Indices=1:n,2:n+1  OutputSizes=1,1
  Assignment2 : Assignment  NumberOfDimensions=2  DiagnosticForDimensions=Warning  IndexOptions=Index vector (dialog),Index vector (dialog)  Indices=1:n,n+2:2*n+1  OutputSizes=1,1
  Constant : Constant  Value=zeros(n,2*n+1)
  Constant1 : Constant  Value=ones(1,n)  VectorParams1D=off
  Gain : Gain  Gain=c_sqrt
  Matrix Multiply : Product  Multiplication=Matrix(*)
  Sum : Sum  Inputs=|++
  Sum1 : Sum  Inputs=|+-
  X0 : Outport
  wires:
  Assignment2/1 -> X0/1
  Assignment1/1 -> Assignment2/1
  Assignment/1 -> Assignment1/1
  Constant/1 -> Assignment/1
  Sum1/1 -> Assignment2/2
  Sum/1 -> Assignment1/2
  Gain/1 -> Sum/2, Sum1/2
  Matrix Multiply/1 -> Sum/1, Sum1/1
  Constant1/1 -> Matrix Multiply/2
  x0/1 -> Assignment/2, Matrix Multiply/1
  A/1 -> Gain/1

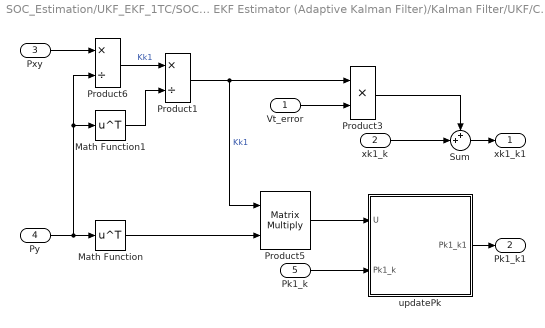
== system SOC_Estimation/UKF_EKF_1TC/SOC EKF Estimator (Adaptive Kalman Filter)/Kalman Filter/UKF/Correction ==
  Vt_error : Inport
  xk1_k : Inport  Port=2
  Pxy : Inport  Port=3
  Py : Inport  Port=4
  Pk1_k : Inport  Port=5
  Math Function : Math  Operator=transpose
  Math Function1 : Math  Operator=transpose
  Product1 : Product  Inputs=*/
  Product3 : Product
  Product5 : Product  Multiplication=Matrix(*)
  Product6 : Product  Inputs=*/
  Sum : Sum  Inputs=++|
  updatePk : MATLAB Function  TreatAsAtomicUnit=on
  xk1_k1 : Outport
  Pk1_k1 : Outport  Port=2
  wires:
  Pk1_k/1 -> updatePk/2(Pk1_k)
  Product5/1 -> updatePk/1(U)
  updatePk/1(Pk1_k1) -> Pk1_k1/1
  Product1/1 -> Product3/1, Product5/1  "Kk1"
  Math Function1/1 -> Product1/2
  Product6/1 -> Product1/1  "Kk1"
  Product3/1 -> Sum/1
  Sum/1 -> xk1_k1/1
  Py/1 -> Math Function/1, Product6/2, Math Function1/1
  Pxy/1 -> Product6/1
  Vt_error/1 -> Product3/2
  xk1_k/1 -> Sum/2
  Math Function/1 -> Product5/2

== system SOC_Estimation/UKF_EKF_1TC/SOC EKF Estimator (Adaptive Kalman Filter)/Kalman Filter/UKF/Delay - X ==
  u : Inport
  SOC0 : Inport  Port=2
  R00 : Inport  Port=3
  Constant1 : Constant  Value=0
  Delay : Delay  DelayLength=1  InitialConditionSource=Input port  SampleTime=Ts
      settings: InputPortMap=u0,p4
  Mux : Mux  Inputs=3
  Reshape : Reshape  OutputDimensionality=Customize  OutputDimensions=[n,1]
  y : Outport
  wires:
  Reshape/1 -> Delay/2
  Constant1/1 -> Mux/2
  SOC0/1 -> Mux/1
  Mux/1 -> Reshape/1
  Delay/1 -> y/1
  u/1 -> Delay/1
  R00/1 -> Mux/3

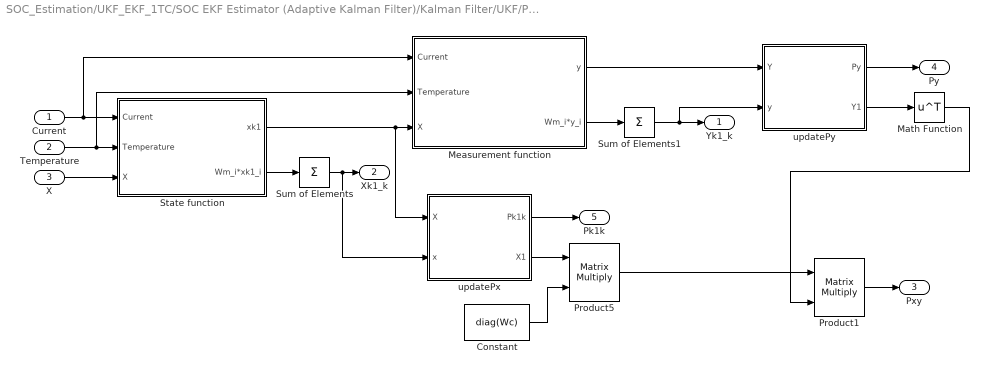
== system SOC_Estimation/UKF_EKF_1TC/SOC EKF Estimator (Adaptive Kalman Filter)/Kalman Filter/UKF/Prediction ==
  Current : Inport
  Temperature : Inport  Port=2
  X : Inport  Port=3
  Constant : Constant  Value=diag(Wc)
  Math Function : Math  Operator=transpose
  Measurement function : Subsystem  TreatAsAtomicUnit=on
  Product1 : Product  Multiplication=Matrix(*)
  Product5 : Product  Multiplication=Matrix(*)
  State function : Subsystem  TreatAsAtomicUnit=on
  Sum of Elements : Sum  Inputs=+  CollapseMode=Specified dimension  CollapseDim=2
  Sum of Elements1 : Sum  Inputs=+  CollapseMode=Specified dimension  CollapseDim=2
  updatePx : MATLAB Function  TreatAsAtomicUnit=on
  updatePy : MATLAB Function  TreatAsAtomicUnit=on
  Yk1_k : Outport
  Xk1_k : Outport  Port=2
  Pxy : Outport  Port=3
  Py : Outport  Port=4
  Pk1k : Outport  Port=5
  wires:
  updatePx/1(Pk1k) -> Pk1k/1
  updatePy/1(Py) -> Py/1
  Product1/1 -> Pxy/1
  Math Function/1 -> Product1/2
  Product5/1 -> Product1/1
  updatePy/2(Y1) -> Math Function/1
  Constant/1 -> Product5/2
  updatePx/2(X1) -> Product5/1
  Measurement function/1(y) -> updatePy/1(Y)
  Sum of Elements/1 -> Xk1_k/1, updatePx/2(x)
  Sum of Elements1/1 -> Yk1_k/1, updatePy/2(y)
  Measurement function/2(Wm_i*y_i) -> Sum of Elements1/1
  State function/1(xk1) -> Measurement function/3(X), updatePx/1(X)
  State function/2(Wm_i*xk1_i) -> Sum of Elements/1
  Temperature/1 -> State function/2(Temperature), Measurement function/2(Temperature)
  X/1 -> State function/3(X)
  Current/1 -> State function/1(Current), Measurement function/1(Current)

== system SOC_Estimation/UKF_EKF_1TC/SOC EKF Estimator (Adaptive Kalman Filter)/Kalman Filter/UKF/Sigma points ==
  x : Inport
  P : Inport  Port=2
  Assignment : Assignment  NumberOfDimensions=2  DiagnosticForDimensions=Warning  IndexOptions=Index vector (dialog),Index vector (dialog)  Indices=1:n,1  OutputSizes=1,1
  Assignment1 : Assignment  NumberOfDimensions=2  DiagnosticForDimensions=Warning  IndexOptions=Index vector (dialog),Index vector (dialog)  Indices=1:n,2:n+1  OutputSizes=1,1
  Assignment2 : Assignment  NumberOfDimensions=2  DiagnosticForDimensions=Warning  IndexOptions=Index vector (dialog),Index vector (dialog)  Indices=1:n,n+2:2*n+1  OutputSizes=1,1
  Constant : Constant  Value=zeros(n,2*n+1)
  Constant1 : Constant  Value=ones(1,n)  VectorParams1D=off
  Gain : Gain  Gain=c_sqrt
  Matrix Multiply : Product  Multiplication=Matrix(*)
  Sum : Sum  Inputs=|++
  Sum1 : Sum  Inputs=|+-
  X : Outport
  wires:
  Assignment2/1 -> X/1
  Assignment1/1 -> Assignment2/1
  Assignment/1 -> Assignment1/1
  Constant/1 -> Assignment/1
  Sum1/1 -> Assignment2/2
  Sum/1 -> Assignment1/2
  Gain/1 -> Sum/2, Sum1/2
  Matrix Multiply/1 -> Sum/1, Sum1/1
  Constant1/1 -> Matrix Multiply/2
  x/1 -> Assignment/2, Matrix Multiply/1
  P/1 -> Gain/1

== system SOC_Estimation/UKF_EKF_1TC/SOC EKF Estimator (Adaptive Kalman Filter)/Kalman Filter/UKBF/Prediction-correction/Measurement function ==
  Current : Inport
  Temperature : Inport  Port=2
  X : Inport  Port=3  Partition=on  PartitionDimension=2  PartitionWidth=1  PartitionOffset=0
  Constant : Constant  Value=Wm
  For Each : ForEach  DisableCoverage=on  ShowIterationIndex=on
  Measurement function : Subsystem
  Product : Product
  Selector : Selector  IndexMode=Zero-based  InputPortWidth=2*n+1  IndexOptions=Index vector (port)  Indices=[1 3]  OutputSizes=1
  h(X) : Outport  ConcatenationDimension=2
  mh : Outport  Port=2  ConcatenationDimension=2
  wires:
  Product/1 -> mh/1
  For Each/1 -> Selector/2
  Selector/1 -> Product/1
  Constant/1 -> Selector/1
  X/1 -> Measurement function/3(x)
  Current/1 -> Measurement function/1(Current)
  Temperature/1 -> Measurement function/2(Temperature)
  Measurement function/1(y) -> h(X)/1, Product/2

== system SOC_Estimation/UKF_EKF_1TC/SOC EKF Estimator (Adaptive Kalman Filter)/Kalman Filter/UKBF/Prediction-correction/State function ==
  Current : Inport
  Temperature : Inport  Port=2
  X : Inport  Port=3  Partition=on  PartitionDimension=2  PartitionWidth=1  PartitionOffset=0
  Constant : Constant  Value=Wm
  For Each : ForEach  DisableCoverage=on  ShowIterationIndex=on
  Product : Product
  Product1 : Product
  Selector : Selector  IndexMode=Zero-based  InputPortWidth=2*n+1  IndexOptions=Index vector (port)  Indices=[1 3]  OutputSizes=1
  State function : Subsystem
  f(X) : Outport  ConcatenationDimension=2
  mf : Outport  Port=2  ConcatenationDimension=2
  mx : Outport  Port=3  ConcatenationDimension=2
  wires:
  Product1/1 -> mx/1
  Product/1 -> mf/1
  For Each/1 -> Selector/2
  Selector/1 -> Product/1, Product1/1
  Constant/1 -> Selector/1
  State function/1(f(x)) -> f(X)/1, Product/2
  Temperature/1 -> State function/2(Temperature)
  Current/1 -> State function/1(Current)
  X/1 -> State function/3(x), Product1/2

== system SOC_Estimation/UKF_EKF_1TC/SOC EKF Estimator (Adaptive Kalman Filter)/Kalman Filter/UKBF/Prediction-correction/Update A ==
  X : Inport
  Constant : Constant  Value=ones(1,2*n+1)  VectorParams1D=off
  Gain : Gain  Gain=1/c_sqrt
  Matrix Multiply : Product  Multiplication=Matrix(*)
  Selector : Selector  NumberOfDimensions=2  InputPortWidth=3  IndexOptions=Index vector (dialog),Index vector (dialog)  Indices=[1:n],1  OutputSizes=1,1
  Selector1 : Selector  NumberOfDimensions=2  InputPortWidth=3  IndexOptions=Index vector (dialog),Index vector (dialog)  Indices=1:n,2:n+1  OutputSizes=1,1
  Sum : Sum  Inputs=|+-
  A(t) : Outport
  xhat : Outport  Port=2
  wires:
  Selector1/1 -> A(t)/1
  Gain/1 -> Selector1/1
  Sum/1 -> Gain/1
  Matrix Multiply/1 -> Sum/2
  Constant/1 -> Matrix Multiply/2
  Selector/1 -> Matrix Multiply/1, xhat/1
  X/1 -> Sum/1, Selector/1

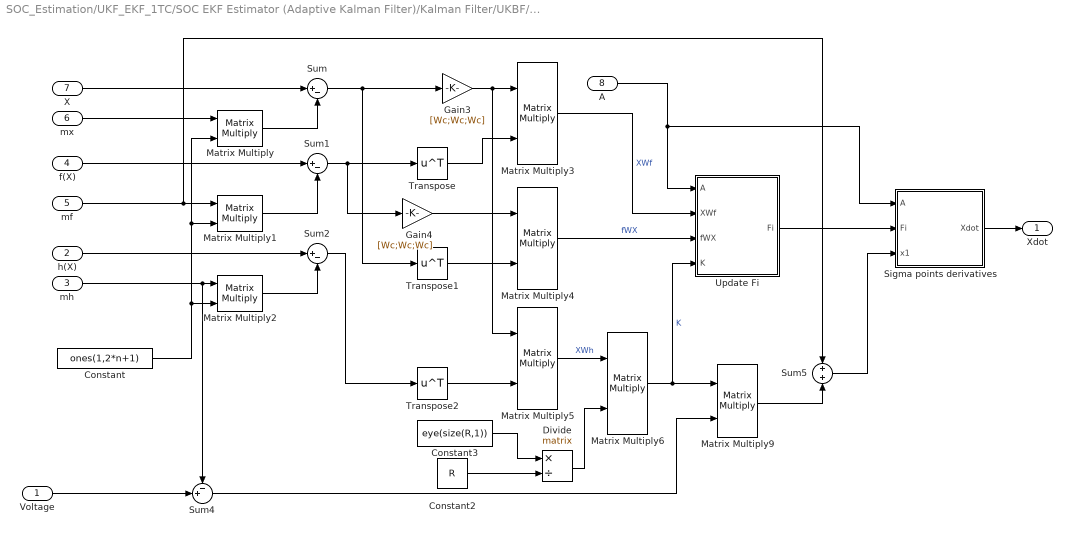
== system SOC_Estimation/UKF_EKF_1TC/SOC EKF Estimator (Adaptive Kalman Filter)/Kalman Filter/UKBF/Prediction-correction/Xdot ==
  Voltage : Inport
  h(X) : Inport  Port=2
  mh : Inport  Port=3
  f(X) : Inport  Port=4
  mf : Inport  Port=5
  mx : Inport  Port=6
  X : Inport  Port=7
  A : Inport  Port=8
  Constant : Constant  Value=ones(1,2*n+1)  VectorParams1D=off
  Constant2 : Constant  Value=R
  Constant3 : Constant  Value=eye(size(R,1))
  Divide : Product  Inputs=*/  Multiplication=Matrix(*)
  Gain3 : Gain  Gain=[Wc;Wc;Wc]
  Gain4 : Gain  Gain=[Wc;Wc;Wc]
  Matrix Multiply{,1..6,9} (8 alike) : Product  Multiplication=Matrix(*)
  Sigma points derivatives : Subsystem
  Sum : Sum  Inputs=|+-
  Sum1 : Sum  Inputs=|+-
  Sum2 : Sum  Inputs=|+-
  Sum4 : Sum  Inputs=-+|
  Sum5 : Sum
  Transpose : Math  Operator=transpose
  Transpose1 : Math  Operator=transpose
  Transpose2 : Math  Operator=transpose
  Update Fi : Subsystem
  Xdot : Outport
  wires:
  Update Fi/1(Fi) -> Sigma points derivatives/2(Fi)
  Sigma points derivatives/1(Xdot) -> Xdot/1
  Matrix Multiply4/1 -> Update Fi/3(fWX)  "fWX"
  Matrix Multiply3/1 -> Update Fi/2(XWf)  "XWf"
  A/1 -> Update Fi/1(A), Sigma points derivatives/1(A)
  Sum5/1 -> Sigma points derivatives/3(x1)
  Matrix Multiply9/1 -> Sum5/2
  Sum4/1 -> Matrix Multiply9/2
  Voltage/1 -> Sum4/2
  Matrix Multiply6/1 -> Matrix Multiply9/1, Update Fi/4(K)  "K"
  Divide/1 -> Matrix Multiply6/2
  Constant3/1 -> Divide/1
  Constant2/1 -> Divide/2
  Matrix Multiply5/1 -> Matrix Multiply6/1  "XWh"
  Transpose2/1 -> Matrix Multiply5/2
  Sum2/1 -> Transpose2/1
  Transpose1/1 -> Matrix Multiply4/2
  Sum/1 -> Gain3/1, Transpose1/1
  Gain4/1 -> Matrix Multiply4/1
  Matrix Multiply2/1 -> Sum2/2
  Gain3/1 -> Matrix Multiply3/1, Matrix Multiply5/1
  Transpose/1 -> Matrix Multiply3/2
  Sum1/1 -> Transpose/1, Gain4/1
  Matrix Multiply1/1 -> Sum1/2
  Matrix Multiply/1 -> Sum/2
  mh/1 -> Matrix Multiply2/1, Sum4/1
  h(X)/1 -> Sum2/1
  mf/1 -> Sum5/1, Matrix Multiply1/1
  f(X)/1 -> Sum1/1
  mx/1 -> Matrix Multiply/1
  X/1 -> Sum/1
  Constant/1 -> Matrix Multiply2/2, Matrix Multiply1/2, Matrix Multiply/2

== system SOC_Estimation/UKF_EKF_1TC/SOC EKF Estimator (Adaptive Kalman Filter)/Kalman Filter/UKF/Prediction/Measurement function ==
  Current : Inport
  Temperature : Inport  Port=2
  X : Inport  Port=3  Partition=on  PartitionDimension=2  PartitionWidth=1  PartitionOffset=0
  Constant : Constant  Value=Wm
  For Each : ForEach  DisableCoverage=on  ShowIterationIndex=on
  Measurement function : Subsystem
  Product : Product
  Selector : Selector  IndexMode=Zero-based  InputPortWidth=2*n+1  IndexOptions=Index vector (port)  Indices=[1 3]  OutputSizes=1
  y : Outport  ConcatenationDimension=2
  Wm_i*y_i : Outport  Port=2  SampleTime=Ts  ConcatenationDimension=2
  wires:
  X/1 -> Measurement function/3(x)
  Current/1 -> Measurement function/1(Current)
  Temperature/1 -> Measurement function/2(Temperature)
  Measurement function/1(y) -> y/1, Product/2
  For Each/1 -> Selector/2
  Constant/1 -> Selector/1
  Selector/1 -> Product/1
  Product/1 -> Wm_i*y_i/1

== system SOC_Estimation/UKF_EKF_1TC/SOC EKF Estimator (Adaptive Kalman Filter)/Kalman Filter/UKF/Prediction/State function ==
  Current : Inport
  Temperature : Inport  Port=2
  X : Inport  Port=3  Partition=on  PartitionDimension=2  PartitionWidth=1  PartitionOffset=0
  Constant : Constant  Value=Wm
  For Each : ForEach  DisableCoverage=on  ShowIterationIndex=on
  Product : Product
  Selector : Selector  IndexMode=Zero-based  InputPortWidth=2*n+1  IndexOptions=Index vector (port)  Indices=[1 3]  OutputSizes=1
  State function : Subsystem
  xk1 : Outport  ConcatenationDimension=2
  Wm_i*xk1_i : Outport  Port=2  SampleTime=Ts  ConcatenationDimension=2
  wires:
  Product/1 -> Wm_i*xk1_i/1
  Selector/1 -> Product/1
  Constant/1 -> Selector/1
  For Each/1 -> Selector/2
  State function/1(xk1) -> xk1/1, Product/2
  Temperature/1 -> State function/2(Temperature)
  Current/1 -> State function/1(Current)
  X/1 -> State function/3(x)

== system SOC_Estimation/UKF_EKF_1TC/SOC EKF Estimator (Adaptive Kalman Filter)/Kalman Filter/UKBF/Prediction-correction/Measurement function/Measurement function ==
  Current : Inport
  Temperature : Inport  Port=2
  x : Inport  Port=3
  Add2 : Sum  Inputs=+--
  Get SOC : Selector  InputPortWidth=3  IndexOptions=Index vector (dialog)  Indices=[1]  OutputSizes=1
  Get SOC2 : Selector  InputPortWidth=3  IndexOptions=Index vector (dialog)  Indices=3  OutputSizes=1
  Get V1 : Selector  InputPortWidth=3  IndexOptions=Index vector (dialog)  Indices=2  OutputSizes=1
  OCV Table : Lookup_n-D  BreakpointsForDimension1=SOC_vec  BreakpointsForDimension2=T_vec  BeginIndexSearchUsingPreviousIndexResult=on  Table=V0_mat  ExtrapMethod=Clip  InternalRulePriority=Speed  RndMeth=Simplest
      settings: InputPortMap=u0,u1
  Product2 : Product
  y : Outport
  wires:
  Temperature/1 -> OCV Table/2
  Get SOC2/1 -> Product2/1
  Add2/1 -> y/1
  Product2/1 -> Add2/2
  Get V1/1 -> Add2/3  "U1"
  Get SOC/1 -> OCV Table/1  "SOC"
  Current/1 -> Product2/2
  OCV Table/1 -> Add2/1
  x/1 -> Get V1/1, Get SOC2/1, Get SOC/1

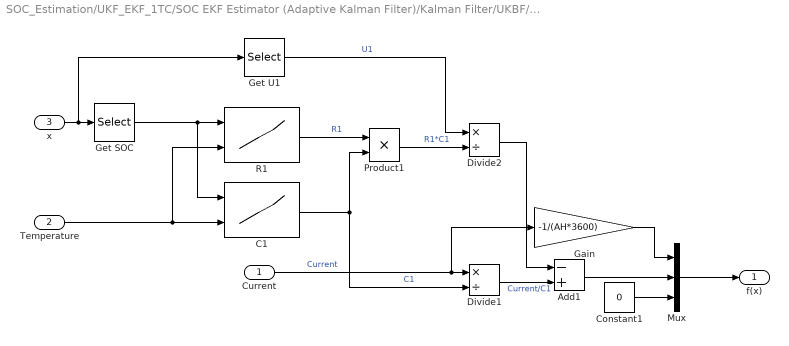
== system SOC_Estimation/UKF_EKF_1TC/SOC EKF Estimator (Adaptive Kalman Filter)/Kalman Filter/UKBF/Prediction-correction/State function/State function ==
  Current : Inport
  Temperature : Inport  Port=2
  x : Inport  Port=3
  Add1 : Sum  Inputs=-+
  C1 : Lookup_n-D  BreakpointsForDimension1=SOC_vec  BreakpointsForDimension2=T_vec  BeginIndexSearchUsingPreviousIndexResult=on  Table=C1_mat  ExtrapMethod=Clip  InternalRulePriority=Speed  RndMeth=Simplest
      settings: InputPortMap=u0,u1
  Constant1 : Constant  Value=0
  Divide1 : Product  Inputs=*/
  Divide2 : Product  Inputs=*/
  Gain : Gain  Gain=-1/(AH*3600)
  Get SOC : Selector  InputPortWidth=3  IndexOptions=Index vector (dialog)  Indices=1  OutputSizes=1
  Get U1 : Selector  InputPortWidth=3  IndexOptions=Index vector (dialog)  Indices=2  OutputSizes=1
  Mux : Mux  Inputs=3
  Product1 : Product
  R1 : Lookup_n-D  BreakpointsForDimension1=SOC_vec  BreakpointsForDimension2=T_vec  BeginIndexSearchUsingPreviousIndexResult=on  Table=R1_mat  ExtrapMethod=Clip  InternalRulePriority=Speed  RndMeth=Simplest
      settings: InputPortMap=u0,u1
  f(x) : Outport
  wires:
  Constant1/1 -> Mux/3
  Divide1/1 -> Add1/2  "Current/C1"
  Product1/1 -> Divide2/2  "R1*C1"
  Get SOC/1 -> C1/1, R1/1
  R1/1 -> Product1/1  "R1"
  Get U1/1 -> Divide2/1  "U1"
  C1/1 -> Product1/2, Divide1/2  "C1"
  Current/1 -> Gain/1, Divide1/1  "Current"
  Mux/1 -> f(x)/1
  Divide2/1 -> Add1/1
  Add1/1 -> Mux/2
  x/1 -> Get U1/1, Get SOC/1
  Temperature/1 -> C1/2, R1/2
  Gain/1 -> Mux/1

== system SOC_Estimation/UKF_EKF_1TC/SOC EKF Estimator (Adaptive Kalman Filter)/Kalman Filter/UKBF/Prediction-correction/Xdot/Sigma points derivatives ==
  A : Inport
  Fi : Inport  Port=2
  x1 : Inport  Port=3
  Assignment : Assignment  NumberOfDimensions=2  DiagnosticForDimensions=Warning  IndexOptions=Index vector (dialog),Index vector (dialog)  Indices=1:n,1  OutputSizes=1,1
  Assignment1 : Assignment  NumberOfDimensions=2  DiagnosticForDimensions=Warning  IndexOptions=Index vector (dialog),Index vector (dialog)  Indices=1:n,2:n+1  OutputSizes=1,1
  Assignment2 : Assignment  NumberOfDimensions=2  DiagnosticForDimensions=Warning  IndexOptions=Index vector (dialog),Index vector (dialog)  Indices=1:n,n+2:2*n+1  OutputSizes=1,1
  Constant : Constant  Value=zeros(n,2*n+1)
  Constant1 : Constant  Value=ones(1,n)  VectorParams1D=off
  Gain : Gain  Gain=c_sqrt
  Matrix Multiply : Product  Multiplication=Matrix(*)
  Matrix Multiply1 : Product  Multiplication=Matrix(*)
  Sum : Sum  Inputs=|++
  Sum1 : Sum  Inputs=|+-
  Xdot : Outport
  wires:
  Matrix Multiply1/1 -> Gain/1
  Fi/1 -> Matrix Multiply1/2
  A/1 -> Matrix Multiply1/1
  Assignment2/1 -> Xdot/1
  Assignment1/1 -> Assignment2/1
  Assignment/1 -> Assignment1/1
  Constant/1 -> Assignment/1
  Sum1/1 -> Assignment2/2
  Sum/1 -> Assignment1/2
  Gain/1 -> Sum/2, Sum1/2
  Matrix Multiply/1 -> Sum/1, Sum1/1
  Constant1/1 -> Matrix Multiply/2
  x1/1 -> Assignment/2, Matrix Multiply/1

== system SOC_Estimation/UKF_EKF_1TC/SOC EKF Estimator (Adaptive Kalman Filter)/Kalman Filter/UKBF/Prediction-correction/Xdot/Update Fi ==
  A : Inport
  XWf : Inport  Port=2
  fWX : Inport  Port=3
  K : Inport  Port=4
  Constant1 : Constant  Value=Q
  Constant4 : Constant  Value=eye(size(P0,1))
  Constant5 : Constant  Value=R
  Divide1 : Product  Inputs=*/  Multiplication=Matrix(*)
  Gain5 : Gain  Gain=tril(ones(n)-diag(0.5*ones(1,n)))
  Matrix Multiply7 : Product  Inputs=3  Multiplication=Matrix(*)
  Matrix Multiply8 : Product  Inputs=3  Multiplication=Matrix(*)
  Sum3 : Sum  Inputs=+++-
  Transpose3 : Math  Operator=transpose
  Transpose4 : Math  Operator=transpose
  Fi : Outport
  wires:
  Gain5/1 -> Fi/1  "Fi"
  fWX/1 -> Sum3/2
  Constant5/1 -> Matrix Multiply8/2
  Transpose4/1 -> Matrix Multiply7/3
  Constant4/1 -> Divide1/1
  XWf/1 -> Sum3/1
  K/1 -> Matrix Multiply8/1, Transpose3/1
  Divide1/1 -> Matrix Multiply7/1, Transpose4/1
  Matrix Multiply8/1 -> Sum3/4
  Transpose3/1 -> Matrix Multiply8/3
  Sum3/1 -> Matrix Multiply7/2
  Constant1/1 -> Sum3/3
  Matrix Multiply7/1 -> Gain5/1  "M"
  A/1 -> Divide1/2

== system SOC_Estimation/UKF_EKF_1TC/SOC EKF Estimator (Adaptive Kalman Filter)/Kalman Filter/UKF/Prediction/Measurement function/Measurement function ==
  Current : Inport
  Temperature : Inport  Port=2
  x : Inport  Port=3
  Add2 : Sum  Inputs=+--
  Get SOC : Selector  InputPortWidth=3  IndexOptions=Index vector (dialog)  Indices=[1]  OutputSizes=1
  Get SOC2 : Selector  InputPortWidth=3  IndexOptions=Index vector (dialog)  Indices=3  OutputSizes=1
  Get V1 : Selector  InputPortWidth=3  IndexOptions=Index vector (dialog)  Indices=2  OutputSizes=1
  OCV Table : Lookup_n-D  BreakpointsForDimension1=SOC_vec  BreakpointsForDimension2=T_vec  BeginIndexSearchUsingPreviousIndexResult=on  Table=V0_mat  ExtrapMethod=Clip  InternalRulePriority=Speed  RndMeth=Simplest
      settings: InputPortMap=u0,u1
  Product2 : Product
  y : Outport
  wires:
  Temperature/1 -> OCV Table/2
  Get SOC2/1 -> Product2/1  "SOC"
  x/1 -> Get SOC/1, Get V1/1, Get SOC2/1
  OCV Table/1 -> Add2/1
  Current/1 -> Product2/2
  Get SOC/1 -> OCV Table/1  "SOC"
  Get V1/1 -> Add2/3  "U1"
  Product2/1 -> Add2/2
  Add2/1 -> y/1
